simulink model "PID_controler"  (R2022b)
settings: Solver=FixedStepAuto  StartTime=0.0  StopTime=10.0  FixedStep=1e-3  MaxStep=1e-3  RelTol=1e-3
(part 2 of 2)

== system PID_controler/pid16/Subsystem2 ==
  In1 : Inport
  Derivative : Derivative
  Gain : Gain  Gain=P
  Gain1 : Gain  Gain=I
  Gain2 : Gain  Gain=D
  Integrator : Integrator
  Sum : Sum  Inputs=+++
  Out1 : Outport
  wires:
  Gain/1 -> Gain2/1, Gain1/1, Sum/1
  Gain1/1 -> Integrator/1
  Integrator/1 -> Sum/2
  Gain2/1 -> Derivative/1
  Derivative/1 -> Sum/3
  Sum/1 -> Out1/1
  In1/1 -> Gain/1

== system PID_controler/pid17/Subsystem ==
  In1 : Inport
  Derivative : Derivative
  Gain : Gain  Gain=P
  Gain1 : Gain  Gain=I
  Gain2 : Gain  Gain=D
  Integrator : Integrator
  Sum : Sum  Inputs=+++
  Out1 : Outport
  wires:
  Gain1/1 -> Integrator/1
  Gain2/1 -> Derivative/1
  Sum/1 -> Out1/1
  Integrator/1 -> Sum/2
  Gain/1 -> Sum/1
  Derivative/1 -> Sum/3
  In1/1 -> Gain/1, Gain2/1, Gain1/1

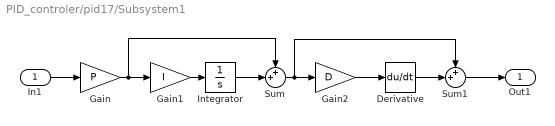
== system PID_controler/pid17/Subsystem1 ==
  In1 : Inport
  Derivative : Derivative
  Gain : Gain  Gain=P
  Gain1 : Gain  Gain=I
  Gain2 : Gain  Gain=D
  Integrator : Integrator
  Sum : Sum  Inputs=++|
  Sum1 : Sum  Inputs=++|
  Out1 : Outport
  wires:
  Sum/1 -> Sum1/1, Gain2/1
  Gain2/1 -> Derivative/1
  Gain/1 -> Sum/1, Gain1/1
  Integrator/1 -> Sum/2
  Gain1/1 -> Integrator/1
  In1/1 -> Gain/1
  Sum1/1 -> Out1/1
  Derivative/1 -> Sum1/2

== system PID_controler/pid17/Subsystem2 ==
  In1 : Inport
  Derivative : Derivative
  Gain : Gain  Gain=P
  Gain1 : Gain  Gain=I
  Gain2 : Gain  Gain=D
  Integrator : Integrator
  Sum : Sum  Inputs=+++
  Out1 : Outport
  wires:
  Gain/1 -> Gain2/1, Gain1/1, Sum/1
  Gain1/1 -> Integrator/1
  Integrator/1 -> Sum/2
  Gain2/1 -> Derivative/1
  Derivative/1 -> Sum/3
  Sum/1 -> Out1/1
  In1/1 -> Gain/1

== system PID_controler/pid18/Subsystem ==
  In1 : Inport
  Derivative : Derivative
  Gain : Gain  Gain=P
  Gain1 : Gain  Gain=I
  Gain2 : Gain  Gain=D
  Integrator : Integrator
  Sum : Sum  Inputs=+++
  Out1 : Outport
  wires:
  Gain1/1 -> Integrator/1
  Gain2/1 -> Derivative/1
  Sum/1 -> Out1/1
  Integrator/1 -> Sum/2
  Gain/1 -> Sum/1
  Derivative/1 -> Sum/3
  In1/1 -> Gain/1, Gain2/1, Gain1/1

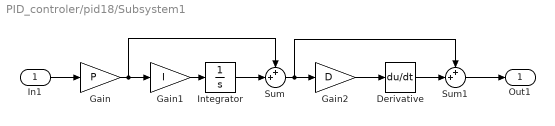
== system PID_controler/pid18/Subsystem1 ==
  In1 : Inport
  Derivative : Derivative
  Gain : Gain  Gain=P
  Gain1 : Gain  Gain=I
  Gain2 : Gain  Gain=D
  Integrator : Integrator
  Sum : Sum  Inputs=++|
  Sum1 : Sum  Inputs=++|
  Out1 : Outport
  wires:
  Sum/1 -> Sum1/1, Gain2/1
  Gain2/1 -> Derivative/1
  Gain/1 -> Sum/1, Gain1/1
  Integrator/1 -> Sum/2
  Gain1/1 -> Integrator/1
  In1/1 -> Gain/1
  Sum1/1 -> Out1/1
  Derivative/1 -> Sum1/2

== system PID_controler/pid18/Subsystem2 ==
  In1 : Inport
  Derivative : Derivative
  Gain : Gain  Gain=P
  Gain1 : Gain  Gain=I
  Gain2 : Gain  Gain=D
  Integrator : Integrator
  Sum : Sum  Inputs=+++
  Out1 : Outport
  wires:
  Gain/1 -> Gain2/1, Gain1/1, Sum/1
  Gain1/1 -> Integrator/1
  Integrator/1 -> Sum/2
  Gain2/1 -> Derivative/1
  Derivative/1 -> Sum/3
  Sum/1 -> Out1/1
  In1/1 -> Gain/1

== system PID_controler/pid19/Subsystem ==
  In1 : Inport
  Derivative : Derivative
  Gain : Gain  Gain=P
  Gain1 : Gain  Gain=I
  Gain2 : Gain  Gain=D
  Integrator : Integrator
  Sum : Sum  Inputs=+++
  Out1 : Outport
  wires:
  Gain1/1 -> Integrator/1
  Gain2/1 -> Derivative/1
  Sum/1 -> Out1/1
  Integrator/1 -> Sum/2
  Gain/1 -> Sum/1
  Derivative/1 -> Sum/3
  In1/1 -> Gain/1, Gain2/1, Gain1/1

== system PID_controler/pid19/Subsystem1 ==
  In1 : Inport
  Derivative : Derivative
  Gain : Gain  Gain=P
  Gain1 : Gain  Gain=I
  Gain2 : Gain  Gain=D
  Integrator : Integrator
  Sum : Sum  Inputs=++|
  Sum1 : Sum  Inputs=++|
  Out1 : Outport
  wires:
  Sum/1 -> Sum1/1, Gain2/1
  Gain2/1 -> Derivative/1
  Gain/1 -> Sum/1, Gain1/1
  Integrator/1 -> Sum/2
  Gain1/1 -> Integrator/1
  In1/1 -> Gain/1
  Sum1/1 -> Out1/1
  Derivative/1 -> Sum1/2

== system PID_controler/pid19/Subsystem2 ==
  In1 : Inport
  Derivative : Derivative
  Gain : Gain  Gain=P
  Gain1 : Gain  Gain=I
  Gain2 : Gain  Gain=D
  Integrator : Integrator
  Sum : Sum  Inputs=+++
  Out1 : Outport
  wires:
  Gain/1 -> Gain2/1, Gain1/1, Sum/1
  Gain1/1 -> Integrator/1
  Integrator/1 -> Sum/2
  Gain2/1 -> Derivative/1
  Derivative/1 -> Sum/3
  Sum/1 -> Out1/1
  In1/1 -> Gain/1

== system PID_controler/pid2/Subsystem ==
  In1 : Inport
  Derivative : Derivative
  Gain : Gain  Gain=P
  Gain1 : Gain  Gain=I
  Gain2 : Gain  Gain=D
  Integrator : Integrator
  Sum : Sum  Inputs=+++
  Out1 : Outport
  wires:
  In1/1 -> Gain1/1, Gain2/1, Gain/1
  Derivative/1 -> Sum/3
  Gain/1 -> Sum/1
  Integrator/1 -> Sum/2
  Sum/1 -> Out1/1
  Gain2/1 -> Derivative/1
  Gain1/1 -> Integrator/1

== system PID_controler/pid2/Subsystem1 ==
  In1 : Inport
  Derivative : Derivative
  Gain : Gain  Gain=P
  Gain1 : Gain  Gain=I
  Gain2 : Gain  Gain=D
  Integrator : Integrator
  Sum : Sum  Inputs=++|
  Sum1 : Sum  Inputs=++|
  Out1 : Outport
  wires:
  Derivative/1 -> Sum1/2
  Sum1/1 -> Out1/1
  In1/1 -> Gain/1
  Gain1/1 -> Integrator/1
  Integrator/1 -> Sum/2
  Gain/1 -> Gain1/1, Sum/1
  Gain2/1 -> Derivative/1
  Sum/1 -> Gain2/1, Sum1/1

== system PID_controler/pid2/Subsystem2 ==
  In1 : Inport
  Derivative : Derivative
  Gain : Gain  Gain=P
  Gain1 : Gain  Gain=I
  Gain2 : Gain  Gain=D
  Integrator : Integrator
  Sum : Sum  Inputs=+++
  Out1 : Outport
  wires:
  In1/1 -> Gain/1
  Sum/1 -> Out1/1
  Derivative/1 -> Sum/3
  Gain2/1 -> Derivative/1
  Integrator/1 -> Sum/2
  Gain1/1 -> Integrator/1
  Gain/1 -> Sum/1, Gain1/1, Gain2/1

== system PID_controler/pid20/Subsystem ==
  In1 : Inport
  Derivative : Derivative
  Gain : Gain  Gain=P
  Gain1 : Gain  Gain=I
  Gain2 : Gain  Gain=D
  Integrator : Integrator
  Sum : Sum  Inputs=+++
  Out1 : Outport
  wires:
  In1/1 -> Gain1/1, Gain2/1, Gain/1
  Derivative/1 -> Sum/3
  Gain/1 -> Sum/1
  Integrator/1 -> Sum/2
  Sum/1 -> Out1/1
  Gain2/1 -> Derivative/1
  Gain1/1 -> Integrator/1

== system PID_controler/pid20/Subsystem1 ==
  In1 : Inport
  Derivative : Derivative
  Gain : Gain  Gain=P
  Gain1 : Gain  Gain=I
  Gain2 : Gain  Gain=D
  Integrator : Integrator
  Sum : Sum  Inputs=++|
  Sum1 : Sum  Inputs=++|
  Out1 : Outport
  wires:
  Derivative/1 -> Sum1/2
  Sum1/1 -> Out1/1
  In1/1 -> Gain/1
  Gain1/1 -> Integrator/1
  Integrator/1 -> Sum/2
  Gain/1 -> Gain1/1, Sum/1
  Gain2/1 -> Derivative/1
  Sum/1 -> Gain2/1, Sum1/1

== system PID_controler/pid20/Subsystem2 ==
  In1 : Inport
  Derivative : Derivative
  Gain : Gain  Gain=P
  Gain1 : Gain  Gain=I
  Gain2 : Gain  Gain=D
  Integrator : Integrator
  Sum : Sum  Inputs=+++
  Out1 : Outport
  wires:
  In1/1 -> Gain/1
  Sum/1 -> Out1/1
  Derivative/1 -> Sum/3
  Gain2/1 -> Derivative/1
  Integrator/1 -> Sum/2
  Gain1/1 -> Integrator/1
  Gain/1 -> Sum/1, Gain1/1, Gain2/1

== system PID_controler/pid21/Subsystem ==
  In1 : Inport
  Derivative : Derivative
  Gain : Gain  Gain=P
  Gain1 : Gain  Gain=I
  Gain2 : Gain  Gain=D
  Integrator : Integrator
  Sum : Sum  Inputs=+++
  Out1 : Outport
  wires:
  In1/1 -> Gain1/1, Gain2/1, Gain/1
  Derivative/1 -> Sum/3
  Gain/1 -> Sum/1
  Integrator/1 -> Sum/2
  Sum/1 -> Out1/1
  Gain2/1 -> Derivative/1
  Gain1/1 -> Integrator/1

== system PID_controler/pid21/Subsystem1 ==
  In1 : Inport
  Derivative : Derivative
  Gain : Gain  Gain=P
  Gain1 : Gain  Gain=I
  Gain2 : Gain  Gain=D
  Integrator : Integrator
  Sum : Sum  Inputs=++|
  Sum1 : Sum  Inputs=++|
  Out1 : Outport
  wires:
  Derivative/1 -> Sum1/2
  Sum1/1 -> Out1/1
  In1/1 -> Gain/1
  Gain1/1 -> Integrator/1
  Integrator/1 -> Sum/2
  Gain/1 -> Gain1/1, Sum/1
  Gain2/1 -> Derivative/1
  Sum/1 -> Gain2/1, Sum1/1

== system PID_controler/pid21/Subsystem2 ==
  In1 : Inport
  Derivative : Derivative
  Gain : Gain  Gain=P
  Gain1 : Gain  Gain=I
  Gain2 : Gain  Gain=D
  Integrator : Integrator
  Sum : Sum  Inputs=+++
  Out1 : Outport
  wires:
  In1/1 -> Gain/1
  Sum/1 -> Out1/1
  Derivative/1 -> Sum/3
  Gain2/1 -> Derivative/1
  Integrator/1 -> Sum/2
  Gain1/1 -> Integrator/1
  Gain/1 -> Sum/1, Gain1/1, Gain2/1

== system PID_controler/pid22/Subsystem ==
  In1 : Inport
  Derivative : Derivative
  Gain : Gain  Gain=P
  Gain1 : Gain  Gain=I
  Gain2 : Gain  Gain=D
  Integrator : Integrator
  Sum : Sum  Inputs=+++
  Out1 : Outport
  wires:
  In1/1 -> Gain1/1, Gain2/1, Gain/1
  Derivative/1 -> Sum/3
  Gain/1 -> Sum/1
  Integrator/1 -> Sum/2
  Sum/1 -> Out1/1
  Gain2/1 -> Derivative/1
  Gain1/1 -> Integrator/1

== system PID_controler/pid22/Subsystem1 ==
  In1 : Inport
  Derivative : Derivative
  Gain : Gain  Gain=P
  Gain1 : Gain  Gain=I
  Gain2 : Gain  Gain=D
  Integrator : Integrator
  Sum : Sum  Inputs=++|
  Sum1 : Sum  Inputs=++|
  Out1 : Outport
  wires:
  Derivative/1 -> Sum1/2
  Sum1/1 -> Out1/1
  In1/1 -> Gain/1
  Gain1/1 -> Integrator/1
  Integrator/1 -> Sum/2
  Gain/1 -> Gain1/1, Sum/1
  Gain2/1 -> Derivative/1
  Sum/1 -> Gain2/1, Sum1/1

== system PID_controler/pid22/Subsystem2 ==
  In1 : Inport
  Derivative : Derivative
  Gain : Gain  Gain=P
  Gain1 : Gain  Gain=I
  Gain2 : Gain  Gain=D
  Integrator : Integrator
  Sum : Sum  Inputs=+++
  Out1 : Outport
  wires:
  In1/1 -> Gain/1
  Sum/1 -> Out1/1
  Derivative/1 -> Sum/3
  Gain2/1 -> Derivative/1
  Integrator/1 -> Sum/2
  Gain1/1 -> Integrator/1
  Gain/1 -> Sum/1, Gain1/1, Gain2/1

== system PID_controler/pid23/Subsystem ==
  In1 : Inport
  Derivative : Derivative
  Gain : Gain  Gain=P
  Gain1 : Gain  Gain=I
  Gain2 : Gain  Gain=D
  Integrator : Integrator
  Sum : Sum  Inputs=+++
  Out1 : Outport
  wires:
  In1/1 -> Gain1/1, Gain2/1, Gain/1
  Derivative/1 -> Sum/3
  Gain/1 -> Sum/1
  Integrator/1 -> Sum/2
  Sum/1 -> Out1/1
  Gain2/1 -> Derivative/1
  Gain1/1 -> Integrator/1

== system PID_controler/pid23/Subsystem1 ==
  In1 : Inport
  Derivative : Derivative
  Gain : Gain  Gain=P
  Gain1 : Gain  Gain=I
  Gain2 : Gain  Gain=D
  Integrator : Integrator
  Sum : Sum  Inputs=++|
  Sum1 : Sum  Inputs=++|
  Out1 : Outport
  wires:
  Derivative/1 -> Sum1/2
  Sum1/1 -> Out1/1
  In1/1 -> Gain/1
  Gain1/1 -> Integrator/1
  Integrator/1 -> Sum/2
  Gain/1 -> Gain1/1, Sum/1
  Gain2/1 -> Derivative/1
  Sum/1 -> Gain2/1, Sum1/1

== system PID_controler/pid23/Subsystem2 ==
  In1 : Inport
  Derivative : Derivative
  Gain : Gain  Gain=P
  Gain1 : Gain  Gain=I
  Gain2 : Gain  Gain=D
  Integrator : Integrator
  Sum : Sum  Inputs=+++
  Out1 : Outport
  wires:
  In1/1 -> Gain/1
  Sum/1 -> Out1/1
  Derivative/1 -> Sum/3
  Gain2/1 -> Derivative/1
  Integrator/1 -> Sum/2
  Gain1/1 -> Integrator/1
  Gain/1 -> Sum/1, Gain1/1, Gain2/1

== system PID_controler/pid24/Subsystem ==
  In1 : Inport
  Derivative : Derivative
  Gain : Gain  Gain=P
  Gain1 : Gain  Gain=I
  Gain2 : Gain  Gain=D
  Integrator : Integrator
  Sum : Sum  Inputs=+++
  Out1 : Outport
  wires:
  In1/1 -> Gain1/1, Gain2/1, Gain/1
  Derivative/1 -> Sum/3
  Gain/1 -> Sum/1
  Integrator/1 -> Sum/2
  Sum/1 -> Out1/1
  Gain2/1 -> Derivative/1
  Gain1/1 -> Integrator/1

== system PID_controler/pid24/Subsystem1 ==
  In1 : Inport
  Derivative : Derivative
  Gain : Gain  Gain=P
  Gain1 : Gain  Gain=I
  Gain2 : Gain  Gain=D
  Integrator : Integrator
  Sum : Sum  Inputs=++|
  Sum1 : Sum  Inputs=++|
  Out1 : Outport
  wires:
  Derivative/1 -> Sum1/2
  Sum1/1 -> Out1/1
  In1/1 -> Gain/1
  Gain1/1 -> Integrator/1
  Integrator/1 -> Sum/2
  Gain/1 -> Gain1/1, Sum/1
  Gain2/1 -> Derivative/1
  Sum/1 -> Gain2/1, Sum1/1

== system PID_controler/pid24/Subsystem2 ==
  In1 : Inport
  Derivative : Derivative
  Gain : Gain  Gain=P
  Gain1 : Gain  Gain=I
  Gain2 : Gain  Gain=D
  Integrator : Integrator
  Sum : Sum  Inputs=+++
  Out1 : Outport
  wires:
  In1/1 -> Gain/1
  Sum/1 -> Out1/1
  Derivative/1 -> Sum/3
  Gain2/1 -> Derivative/1
  Integrator/1 -> Sum/2
  Gain1/1 -> Integrator/1
  Gain/1 -> Sum/1, Gain1/1, Gain2/1

== system PID_controler/pid25/Subsystem ==
  In1 : Inport
  Derivative : Derivative
  Gain : Gain  Gain=P
  Gain1 : Gain  Gain=I
  Gain2 : Gain  Gain=D
  Integrator : Integrator
  Sum : Sum  Inputs=+++
  Out1 : Outport
  wires:
  In1/1 -> Gain1/1, Gain2/1, Gain/1
  Derivative/1 -> Sum/3
  Gain/1 -> Sum/1
  Integrator/1 -> Sum/2
  Sum/1 -> Out1/1
  Gain2/1 -> Derivative/1
  Gain1/1 -> Integrator/1

== system PID_controler/pid25/Subsystem1 ==
  In1 : Inport
  Derivative : Derivative
  Gain : Gain  Gain=P
  Gain1 : Gain  Gain=I
  Gain2 : Gain  Gain=D
  Integrator : Integrator
  Sum : Sum  Inputs=++|
  Sum1 : Sum  Inputs=++|
  Out1 : Outport
  wires:
  Derivative/1 -> Sum1/2
  Sum1/1 -> Out1/1
  In1/1 -> Gain/1
  Gain1/1 -> Integrator/1
  Integrator/1 -> Sum/2
  Gain/1 -> Gain1/1, Sum/1
  Gain2/1 -> Derivative/1
  Sum/1 -> Gain2/1, Sum1/1

== system PID_controler/pid25/Subsystem2 ==
  In1 : Inport
  Derivative : Derivative
  Gain : Gain  Gain=P
  Gain1 : Gain  Gain=I
  Gain2 : Gain  Gain=D
  Integrator : Integrator
  Sum : Sum  Inputs=+++
  Out1 : Outport
  wires:
  In1/1 -> Gain/1
  Sum/1 -> Out1/1
  Derivative/1 -> Sum/3
  Gain2/1 -> Derivative/1
  Integrator/1 -> Sum/2
  Gain1/1 -> Integrator/1
  Gain/1 -> Sum/1, Gain1/1, Gain2/1

== system PID_controler/pid26/Subsystem ==
  In1 : Inport
  Derivative : Derivative
  Gain : Gain  Gain=P
  Gain1 : Gain  Gain=I
  Gain2 : Gain  Gain=D
  Integrator : Integrator
  Sum : Sum  Inputs=+++
  Out1 : Outport
  wires:
  In1/1 -> Gain1/1, Gain2/1, Gain/1
  Derivative/1 -> Sum/3
  Gain/1 -> Sum/1
  Integrator/1 -> Sum/2
  Sum/1 -> Out1/1
  Gain2/1 -> Derivative/1
  Gain1/1 -> Integrator/1

== system PID_controler/pid26/Subsystem1 ==
  In1 : Inport
  Derivative : Derivative
  Gain : Gain  Gain=P
  Gain1 : Gain  Gain=I
  Gain2 : Gain  Gain=D
  Integrator : Integrator
  Sum : Sum  Inputs=++|
  Sum1 : Sum  Inputs=++|
  Out1 : Outport
  wires:
  Derivative/1 -> Sum1/2
  Sum1/1 -> Out1/1
  In1/1 -> Gain/1
  Gain1/1 -> Integrator/1
  Integrator/1 -> Sum/2
  Gain/1 -> Gain1/1, Sum/1
  Gain2/1 -> Derivative/1
  Sum/1 -> Gain2/1, Sum1/1

== system PID_controler/pid26/Subsystem2 ==
  In1 : Inport
  Derivative : Derivative
  Gain : Gain  Gain=P
  Gain1 : Gain  Gain=I
  Gain2 : Gain  Gain=D
  Integrator : Integrator
  Sum : Sum  Inputs=+++
  Out1 : Outport
  wires:
  In1/1 -> Gain/1
  Sum/1 -> Out1/1
  Derivative/1 -> Sum/3
  Gain2/1 -> Derivative/1
  Integrator/1 -> Sum/2
  Gain1/1 -> Integrator/1
  Gain/1 -> Sum/1, Gain1/1, Gain2/1

== system PID_controler/pid27/Subsystem ==
  In1 : Inport
  Derivative : Derivative
  Gain : Gain  Gain=P
  Gain1 : Gain  Gain=I
  Gain2 : Gain  Gain=D
  Integrator : Integrator
  Sum : Sum  Inputs=+++
  Out1 : Outport
  wires:
  In1/1 -> Gain1/1, Gain2/1, Gain/1
  Derivative/1 -> Sum/3
  Gain/1 -> Sum/1
  Integrator/1 -> Sum/2
  Sum/1 -> Out1/1
  Gain2/1 -> Derivative/1
  Gain1/1 -> Integrator/1

== system PID_controler/pid27/Subsystem1 ==
  In1 : Inport
  Derivative : Derivative
  Gain : Gain  Gain=P
  Gain1 : Gain  Gain=I
  Gain2 : Gain  Gain=D
  Integrator : Integrator
  Sum : Sum  Inputs=++|
  Sum1 : Sum  Inputs=++|
  Out1 : Outport
  wires:
  Derivative/1 -> Sum1/2
  Sum1/1 -> Out1/1
  In1/1 -> Gain/1
  Gain1/1 -> Integrator/1
  Integrator/1 -> Sum/2
  Gain/1 -> Gain1/1, Sum/1
  Gain2/1 -> Derivative/1
  Sum/1 -> Gain2/1, Sum1/1

== system PID_controler/pid27/Subsystem2 ==
  In1 : Inport
  Derivative : Derivative
  Gain : Gain  Gain=P
  Gain1 : Gain  Gain=I
  Gain2 : Gain  Gain=D
  Integrator : Integrator
  Sum : Sum  Inputs=+++
  Out1 : Outport
  wires:
  In1/1 -> Gain/1
  Sum/1 -> Out1/1
  Derivative/1 -> Sum/3
  Gain2/1 -> Derivative/1
  Integrator/1 -> Sum/2
  Gain1/1 -> Integrator/1
  Gain/1 -> Sum/1, Gain1/1, Gain2/1

== system PID_controler/pid28/Subsystem ==
  In1 : Inport
  Derivative : Derivative
  Gain : Gain  Gain=P
  Gain1 : Gain  Gain=I
  Gain2 : Gain  Gain=D
  Integrator : Integrator
  Sum : Sum  Inputs=+++
  Out1 : Outport
  wires:
  In1/1 -> Gain1/1, Gain2/1, Gain/1
  Derivative/1 -> Sum/3
  Gain/1 -> Sum/1
  Integrator/1 -> Sum/2
  Sum/1 -> Out1/1
  Gain2/1 -> Derivative/1
  Gain1/1 -> Integrator/1

== system PID_controler/pid28/Subsystem1 ==
  In1 : Inport
  Derivative : Derivative
  Gain : Gain  Gain=P
  Gain1 : Gain  Gain=I
  Gain2 : Gain  Gain=D
  Integrator : Integrator
  Sum : Sum  Inputs=++|
  Sum1 : Sum  Inputs=++|
  Out1 : Outport
  wires:
  Derivative/1 -> Sum1/2
  Sum1/1 -> Out1/1
  In1/1 -> Gain/1
  Gain1/1 -> Integrator/1
  Integrator/1 -> Sum/2
  Gain/1 -> Gain1/1, Sum/1
  Gain2/1 -> Derivative/1
  Sum/1 -> Gain2/1, Sum1/1

== system PID_controler/pid28/Subsystem2 ==
  In1 : Inport
  Derivative : Derivative
  Gain : Gain  Gain=P
  Gain1 : Gain  Gain=I
  Gain2 : Gain  Gain=D
  Integrator : Integrator
  Sum : Sum  Inputs=+++
  Out1 : Outport
  wires:
  In1/1 -> Gain/1
  Sum/1 -> Out1/1
  Derivative/1 -> Sum/3
  Gain2/1 -> Derivative/1
  Integrator/1 -> Sum/2
  Gain1/1 -> Integrator/1
  Gain/1 -> Sum/1, Gain1/1, Gain2/1

== system PID_controler/pid29/Subsystem ==
  In1 : Inport
  Derivative : Derivative
  Gain : Gain  Gain=P
  Gain1 : Gain  Gain=I
  Gain2 : Gain  Gain=D
  Integrator : Integrator
  Sum : Sum  Inputs=+++
  Out1 : Outport
  wires:
  In1/1 -> Gain1/1, Gain2/1, Gain/1
  Derivative/1 -> Sum/3
  Gain/1 -> Sum/1
  Integrator/1 -> Sum/2
  Sum/1 -> Out1/1
  Gain2/1 -> Derivative/1
  Gain1/1 -> Integrator/1

== system PID_controler/pid29/Subsystem1 ==
  In1 : Inport
  Derivative : Derivative
  Gain : Gain  Gain=P
  Gain1 : Gain  Gain=I
  Gain2 : Gain  Gain=D
  Integrator : Integrator
  Sum : Sum  Inputs=++|
  Sum1 : Sum  Inputs=++|
  Out1 : Outport
  wires:
  Derivative/1 -> Sum1/2
  Sum1/1 -> Out1/1
  In1/1 -> Gain/1
  Gain1/1 -> Integrator/1
  Integrator/1 -> Sum/2
  Gain/1 -> Gain1/1, Sum/1
  Gain2/1 -> Derivative/1
  Sum/1 -> Gain2/1, Sum1/1

== system PID_controler/pid29/Subsystem2 ==
  In1 : Inport
  Derivative : Derivative
  Gain : Gain  Gain=P
  Gain1 : Gain  Gain=I
  Gain2 : Gain  Gain=D
  Integrator : Integrator
  Sum : Sum  Inputs=+++
  Out1 : Outport
  wires:
  In1/1 -> Gain/1
  Sum/1 -> Out1/1
  Derivative/1 -> Sum/3
  Gain2/1 -> Derivative/1
  Integrator/1 -> Sum/2
  Gain1/1 -> Integrator/1
  Gain/1 -> Sum/1, Gain1/1, Gain2/1

== system PID_controler/pid3/Subsystem ==
  In1 : Inport
  Derivative : Derivative
  Gain : Gain  Gain=P
  Gain1 : Gain  Gain=I
  Gain2 : Gain  Gain=D
  Integrator : Integrator
  Sum : Sum  Inputs=+++
  Out1 : Outport
  wires:
  In1/1 -> Gain1/1, Gain2/1, Gain/1
  Derivative/1 -> Sum/3
  Gain/1 -> Sum/1
  Integrator/1 -> Sum/2
  Sum/1 -> Out1/1
  Gain2/1 -> Derivative/1
  Gain1/1 -> Integrator/1

== system PID_controler/pid3/Subsystem1 ==
  In1 : Inport
  Derivative : Derivative
  Gain : Gain  Gain=P
  Gain1 : Gain  Gain=I
  Gain2 : Gain  Gain=D
  Integrator : Integrator
  Sum : Sum  Inputs=++|
  Sum1 : Sum  Inputs=++|
  Out1 : Outport
  wires:
  Derivative/1 -> Sum1/2
  Sum1/1 -> Out1/1
  In1/1 -> Gain/1
  Gain1/1 -> Integrator/1
  Integrator/1 -> Sum/2
  Gain/1 -> Gain1/1, Sum/1
  Gain2/1 -> Derivative/1
  Sum/1 -> Gain2/1, Sum1/1

== system PID_controler/pid3/Subsystem2 ==
  In1 : Inport
  Derivative : Derivative
  Gain : Gain  Gain=P
  Gain1 : Gain  Gain=I
  Gain2 : Gain  Gain=D
  Integrator : Integrator
  Sum : Sum  Inputs=+++
  Out1 : Outport
  wires:
  In1/1 -> Gain/1
  Sum/1 -> Out1/1
  Derivative/1 -> Sum/3
  Gain2/1 -> Derivative/1
  Integrator/1 -> Sum/2
  Gain1/1 -> Integrator/1
  Gain/1 -> Sum/1, Gain1/1, Gain2/1

== system PID_controler/pid30/Subsystem ==
  In1 : Inport
  Derivative : Derivative
  Gain : Gain  Gain=P
  Gain1 : Gain  Gain=I
  Gain2 : Gain  Gain=D
  Integrator : Integrator
  Sum : Sum  Inputs=+++
  Out1 : Outport
  wires:
  Gain1/1 -> Integrator/1
  Gain2/1 -> Derivative/1
  Sum/1 -> Out1/1
  Integrator/1 -> Sum/2
  Gain/1 -> Sum/1
  Derivative/1 -> Sum/3
  In1/1 -> Gain/1, Gain2/1, Gain1/1

== system PID_controler/pid30/Subsystem1 ==
  In1 : Inport
  Derivative : Derivative
  Gain : Gain  Gain=P
  Gain1 : Gain  Gain=I
  Gain2 : Gain  Gain=D
  Integrator : Integrator
  Sum : Sum  Inputs=++|
  Sum1 : Sum  Inputs=++|
  Out1 : Outport
  wires:
  Sum/1 -> Sum1/1, Gain2/1
  Gain2/1 -> Derivative/1
  Gain/1 -> Sum/1, Gain1/1
  Integrator/1 -> Sum/2
  Gain1/1 -> Integrator/1
  In1/1 -> Gain/1
  Sum1/1 -> Out1/1
  Derivative/1 -> Sum1/2

== system PID_controler/pid30/Subsystem2 ==
  In1 : Inport
  Derivative : Derivative
  Gain : Gain  Gain=P
  Gain1 : Gain  Gain=I
  Gain2 : Gain  Gain=D
  Integrator : Integrator
  Sum : Sum  Inputs=+++
  Out1 : Outport
  wires:
  Gain/1 -> Gain2/1, Gain1/1, Sum/1
  Gain1/1 -> Integrator/1
  Integrator/1 -> Sum/2
  Gain2/1 -> Derivative/1
  Derivative/1 -> Sum/3
  Sum/1 -> Out1/1
  In1/1 -> Gain/1

== system PID_controler/pid31/Subsystem ==
  In1 : Inport
  Derivative : Derivative
  Gain : Gain  Gain=P
  Gain1 : Gain  Gain=I
  Gain2 : Gain  Gain=D
  Integrator : Integrator
  Sum : Sum  Inputs=+++
  Out1 : Outport
  wires:
  Gain1/1 -> Integrator/1
  Gain2/1 -> Derivative/1
  Sum/1 -> Out1/1
  Integrator/1 -> Sum/2
  Gain/1 -> Sum/1
  Derivative/1 -> Sum/3
  In1/1 -> Gain/1, Gain2/1, Gain1/1

== system PID_controler/pid31/Subsystem1 ==
  In1 : Inport
  Derivative : Derivative
  Gain : Gain  Gain=P
  Gain1 : Gain  Gain=I
  Gain2 : Gain  Gain=D
  Integrator : Integrator
  Sum : Sum  Inputs=++|
  Sum1 : Sum  Inputs=++|
  Out1 : Outport
  wires:
  Sum/1 -> Sum1/1, Gain2/1
  Gain2/1 -> Derivative/1
  Gain/1 -> Sum/1, Gain1/1
  Integrator/1 -> Sum/2
  Gain1/1 -> Integrator/1
  In1/1 -> Gain/1
  Sum1/1 -> Out1/1
  Derivative/1 -> Sum1/2

== system PID_controler/pid31/Subsystem2 ==
  In1 : Inport
  Derivative : Derivative
  Gain : Gain  Gain=P
  Gain1 : Gain  Gain=I
  Gain2 : Gain  Gain=D
  Integrator : Integrator
  Sum : Sum  Inputs=+++
  Out1 : Outport
  wires:
  Gain/1 -> Gain2/1, Gain1/1, Sum/1
  Gain1/1 -> Integrator/1
  Integrator/1 -> Sum/2
  Gain2/1 -> Derivative/1
  Derivative/1 -> Sum/3
  Sum/1 -> Out1/1
  In1/1 -> Gain/1

== system PID_controler/pid32/Subsystem ==
  In1 : Inport
  Derivative : Derivative
  Gain : Gain  Gain=P
  Gain1 : Gain  Gain=I
  Gain2 : Gain  Gain=D
  Integrator : Integrator
  Sum : Sum  Inputs=+++
  Out1 : Outport
  wires:
  Gain1/1 -> Integrator/1
  Gain2/1 -> Derivative/1
  Sum/1 -> Out1/1
  Integrator/1 -> Sum/2
  Gain/1 -> Sum/1
  Derivative/1 -> Sum/3
  In1/1 -> Gain/1, Gain2/1, Gain1/1

== system PID_controler/pid32/Subsystem1 ==
  In1 : Inport
  Derivative : Derivative
  Gain : Gain  Gain=P
  Gain1 : Gain  Gain=I
  Gain2 : Gain  Gain=D
  Integrator : Integrator
  Sum : Sum  Inputs=++|
  Sum1 : Sum  Inputs=++|
  Out1 : Outport
  wires:
  Sum/1 -> Sum1/1, Gain2/1
  Gain2/1 -> Derivative/1
  Gain/1 -> Sum/1, Gain1/1
  Integrator/1 -> Sum/2
  Gain1/1 -> Integrator/1
  In1/1 -> Gain/1
  Sum1/1 -> Out1/1
  Derivative/1 -> Sum1/2

== system PID_controler/pid32/Subsystem2 ==
  In1 : Inport
  Derivative : Derivative
  Gain : Gain  Gain=P
  Gain1 : Gain  Gain=I
  Gain2 : Gain  Gain=D
  Integrator : Integrator
  Sum : Sum  Inputs=+++
  Out1 : Outport
  wires:
  Gain/1 -> Gain2/1, Gain1/1, Sum/1
  Gain1/1 -> Integrator/1
  Integrator/1 -> Sum/2
  Gain2/1 -> Derivative/1
  Derivative/1 -> Sum/3
  Sum/1 -> Out1/1
  In1/1 -> Gain/1

== system PID_controler/pid33/Subsystem ==
  In1 : Inport
  Derivative : Derivative
  Gain : Gain  Gain=P
  Gain1 : Gain  Gain=I
  Gain2 : Gain  Gain=D
  Integrator : Integrator
  Sum : Sum  Inputs=+++
  Out1 : Outport
  wires:
  Gain1/1 -> Integrator/1
  Gain2/1 -> Derivative/1
  Sum/1 -> Out1/1
  Integrator/1 -> Sum/2
  Gain/1 -> Sum/1
  Derivative/1 -> Sum/3
  In1/1 -> Gain/1, Gain2/1, Gain1/1

== system PID_controler/pid33/Subsystem1 ==
  In1 : Inport
  Derivative : Derivative
  Gain : Gain  Gain=P
  Gain1 : Gain  Gain=I
  Gain2 : Gain  Gain=D
  Integrator : Integrator
  Sum : Sum  Inputs=++|
  Sum1 : Sum  Inputs=++|
  Out1 : Outport
  wires:
  Sum/1 -> Sum1/1, Gain2/1
  Gain2/1 -> Derivative/1
  Gain/1 -> Sum/1, Gain1/1
  Integrator/1 -> Sum/2
  Gain1/1 -> Integrator/1
  In1/1 -> Gain/1
  Sum1/1 -> Out1/1
  Derivative/1 -> Sum1/2

== system PID_controler/pid33/Subsystem2 ==
  In1 : Inport
  Derivative : Derivative
  Gain : Gain  Gain=P
  Gain1 : Gain  Gain=I
  Gain2 : Gain  Gain=D
  Integrator : Integrator
  Sum : Sum  Inputs=+++
  Out1 : Outport
  wires:
  Gain/1 -> Gain2/1, Gain1/1, Sum/1
  Gain1/1 -> Integrator/1
  Integrator/1 -> Sum/2
  Gain2/1 -> Derivative/1
  Derivative/1 -> Sum/3
  Sum/1 -> Out1/1
  In1/1 -> Gain/1

== system PID_controler/pid34/Subsystem ==
  In1 : Inport
  Derivative : Derivative
  Gain : Gain  Gain=P
  Gain1 : Gain  Gain=I
  Gain2 : Gain  Gain=D
  Integrator : Integrator
  Sum : Sum  Inputs=+++
  Out1 : Outport
  wires:
  Gain1/1 -> Integrator/1
  Gain2/1 -> Derivative/1
  Sum/1 -> Out1/1
  Integrator/1 -> Sum/2
  Gain/1 -> Sum/1
  Derivative/1 -> Sum/3
  In1/1 -> Gain/1, Gain2/1, Gain1/1

== system PID_controler/pid34/Subsystem1 ==
  In1 : Inport
  Derivative : Derivative
  Gain : Gain  Gain=P
  Gain1 : Gain  Gain=I
  Gain2 : Gain  Gain=D
  Integrator : Integrator
  Sum : Sum  Inputs=++|
  Sum1 : Sum  Inputs=++|
  Out1 : Outport
  wires:
  Sum/1 -> Sum1/1, Gain2/1
  Gain2/1 -> Derivative/1
  Gain/1 -> Sum/1, Gain1/1
  Integrator/1 -> Sum/2
  Gain1/1 -> Integrator/1
  In1/1 -> Gain/1
  Sum1/1 -> Out1/1
  Derivative/1 -> Sum1/2

== system PID_controler/pid34/Subsystem2 ==
  In1 : Inport
  Derivative : Derivative
  Gain : Gain  Gain=P
  Gain1 : Gain  Gain=I
  Gain2 : Gain  Gain=D
  Integrator : Integrator
  Sum : Sum  Inputs=+++
  Out1 : Outport
  wires:
  Gain/1 -> Gain2/1, Gain1/1, Sum/1
  Gain1/1 -> Integrator/1
  Integrator/1 -> Sum/2
  Gain2/1 -> Derivative/1
  Derivative/1 -> Sum/3
  Sum/1 -> Out1/1
  In1/1 -> Gain/1

== system PID_controler/pid4/Subsystem ==
  In1 : Inport
  Derivative : Derivative
  Gain : Gain  Gain=P
  Gain1 : Gain  Gain=I
  Gain2 : Gain  Gain=D
  Integrator : Integrator
  Sum : Sum  Inputs=+++
  Out1 : Outport
  wires:
  In1/1 -> Gain1/1, Gain2/1, Gain/1
  Derivative/1 -> Sum/3
  Gain/1 -> Sum/1
  Integrator/1 -> Sum/2
  Sum/1 -> Out1/1
  Gain2/1 -> Derivative/1
  Gain1/1 -> Integrator/1

== system PID_controler/pid4/Subsystem1 ==
  In1 : Inport
  Derivative : Derivative
  Gain : Gain  Gain=P
  Gain1 : Gain  Gain=I
  Gain2 : Gain  Gain=D
  Integrator : Integrator
  Sum : Sum  Inputs=++|
  Sum1 : Sum  Inputs=++|
  Out1 : Outport
  wires:
  Derivative/1 -> Sum1/2
  Sum1/1 -> Out1/1
  In1/1 -> Gain/1
  Gain1/1 -> Integrator/1
  Integrator/1 -> Sum/2
  Gain/1 -> Gain1/1, Sum/1
  Gain2/1 -> Derivative/1
  Sum/1 -> Gain2/1, Sum1/1

== system PID_controler/pid4/Subsystem2 ==
  In1 : Inport
  Derivative : Derivative
  Gain : Gain  Gain=P
  Gain1 : Gain  Gain=I
  Gain2 : Gain  Gain=D
  Integrator : Integrator
  Sum : Sum  Inputs=+++
  Out1 : Outport
  wires:
  In1/1 -> Gain/1
  Sum/1 -> Out1/1
  Derivative/1 -> Sum/3
  Gain2/1 -> Derivative/1
  Integrator/1 -> Sum/2
  Gain1/1 -> Integrator/1
  Gain/1 -> Sum/1, Gain1/1, Gain2/1

== system PID_controler/pid5/Subsystem ==
  In1 : Inport
  Derivative : Derivative
  Gain : Gain  Gain=P
  Gain1 : Gain  Gain=I
  Gain2 : Gain  Gain=D
  Integrator : Integrator
  Sum : Sum  Inputs=+++
  Out1 : Outport
  wires:
  In1/1 -> Gain1/1, Gain2/1, Gain/1
  Derivative/1 -> Sum/3
  Gain/1 -> Sum/1
  Integrator/1 -> Sum/2
  Sum/1 -> Out1/1
  Gain2/1 -> Derivative/1
  Gain1/1 -> Integrator/1

== system PID_controler/pid5/Subsystem1 ==
  In1 : Inport
  Derivative : Derivative
  Gain : Gain  Gain=P
  Gain1 : Gain  Gain=I
  Gain2 : Gain  Gain=D
  Integrator : Integrator
  Sum : Sum  Inputs=++|
  Sum1 : Sum  Inputs=++|
  Out1 : Outport
  wires:
  Derivative/1 -> Sum1/2
  Sum1/1 -> Out1/1
  In1/1 -> Gain/1
  Gain1/1 -> Integrator/1
  Integrator/1 -> Sum/2
  Gain/1 -> Gain1/1, Sum/1
  Gain2/1 -> Derivative/1
  Sum/1 -> Gain2/1, Sum1/1

== system PID_controler/pid5/Subsystem2 ==
  In1 : Inport
  Derivative : Derivative
  Gain : Gain  Gain=P
  Gain1 : Gain  Gain=I
  Gain2 : Gain  Gain=D
  Integrator : Integrator
  Sum : Sum  Inputs=+++
  Out1 : Outport
  wires:
  In1/1 -> Gain/1
  Sum/1 -> Out1/1
  Derivative/1 -> Sum/3
  Gain2/1 -> Derivative/1
  Integrator/1 -> Sum/2
  Gain1/1 -> Integrator/1
  Gain/1 -> Sum/1, Gain1/1, Gain2/1

== system PID_controler/pid6/Subsystem ==
  In1 : Inport
  Derivative : Derivative
  Gain : Gain  Gain=P
  Gain1 : Gain  Gain=I
  Gain2 : Gain  Gain=D
  Integrator : Integrator
  Sum : Sum  Inputs=+++
  Out1 : Outport
  wires:
  In1/1 -> Gain1/1, Gain2/1, Gain/1
  Derivative/1 -> Sum/3
  Gain/1 -> Sum/1
  Integrator/1 -> Sum/2
  Sum/1 -> Out1/1
  Gain2/1 -> Derivative/1
  Gain1/1 -> Integrator/1

== system PID_controler/pid6/Subsystem1 ==
  In1 : Inport
  Derivative : Derivative
  Gain : Gain  Gain=P
  Gain1 : Gain  Gain=I
  Gain2 : Gain  Gain=D
  Integrator : Integrator
  Sum : Sum  Inputs=++|
  Sum1 : Sum  Inputs=++|
  Out1 : Outport
  wires:
  Derivative/1 -> Sum1/2
  Sum1/1 -> Out1/1
  In1/1 -> Gain/1
  Gain1/1 -> Integrator/1
  Integrator/1 -> Sum/2
  Gain/1 -> Gain1/1, Sum/1
  Gain2/1 -> Derivative/1
  Sum/1 -> Gain2/1, Sum1/1

== system PID_controler/pid6/Subsystem2 ==
  In1 : Inport
  Derivative : Derivative
  Gain : Gain  Gain=P
  Gain1 : Gain  Gain=I
  Gain2 : Gain  Gain=D
  Integrator : Integrator
  Sum : Sum  Inputs=+++
  Out1 : Outport
  wires:
  In1/1 -> Gain/1
  Sum/1 -> Out1/1
  Derivative/1 -> Sum/3
  Gain2/1 -> Derivative/1
  Integrator/1 -> Sum/2
  Gain1/1 -> Integrator/1
  Gain/1 -> Sum/1, Gain1/1, Gain2/1

== system PID_controler/pid7/Subsystem ==
  In1 : Inport
  Derivative : Derivative
  Gain : Gain  Gain=P
  Gain1 : Gain  Gain=I
  Gain2 : Gain  Gain=D
  Integrator : Integrator
  Sum : Sum  Inputs=+++
  Out1 : Outport
  wires:
  In1/1 -> Gain1/1, Gain2/1, Gain/1
  Derivative/1 -> Sum/3
  Gain/1 -> Sum/1
  Integrator/1 -> Sum/2
  Sum/1 -> Out1/1
  Gain2/1 -> Derivative/1
  Gain1/1 -> Integrator/1

== system PID_controler/pid7/Subsystem1 ==
  In1 : Inport
  Derivative : Derivative
  Gain : Gain  Gain=P
  Gain1 : Gain  Gain=I
  Gain2 : Gain  Gain=D
  Integrator : Integrator
  Sum : Sum  Inputs=++|
  Sum1 : Sum  Inputs=++|
  Out1 : Outport
  wires:
  Derivative/1 -> Sum1/2
  Sum1/1 -> Out1/1
  In1/1 -> Gain/1
  Gain1/1 -> Integrator/1
  Integrator/1 -> Sum/2
  Gain/1 -> Gain1/1, Sum/1
  Gain2/1 -> Derivative/1
  Sum/1 -> Gain2/1, Sum1/1

== system PID_controler/pid7/Subsystem2 ==
  In1 : Inport
  Derivative : Derivative
  Gain : Gain  Gain=P
  Gain1 : Gain  Gain=I
  Gain2 : Gain  Gain=D
  Integrator : Integrator
  Sum : Sum  Inputs=+++
  Out1 : Outport
  wires:
  In1/1 -> Gain/1
  Sum/1 -> Out1/1
  Derivative/1 -> Sum/3
  Gain2/1 -> Derivative/1
  Integrator/1 -> Sum/2
  Gain1/1 -> Integrator/1
  Gain/1 -> Sum/1, Gain1/1, Gain2/1

== system PID_controler/pid8/Subsystem ==
  In1 : Inport
  Derivative : Derivative
  Gain : Gain  Gain=P
  Gain1 : Gain  Gain=I
  Gain2 : Gain  Gain=D
  Integrator : Integrator
  Sum : Sum  Inputs=+++
  Out1 : Outport
  wires:
  In1/1 -> Gain1/1, Gain2/1, Gain/1
  Derivative/1 -> Sum/3
  Gain/1 -> Sum/1
  Integrator/1 -> Sum/2
  Sum/1 -> Out1/1
  Gain2/1 -> Derivative/1
  Gain1/1 -> Integrator/1

== system PID_controler/pid8/Subsystem1 ==
  In1 : Inport
  Derivative : Derivative
  Gain : Gain  Gain=P
  Gain1 : Gain  Gain=I
  Gain2 : Gain  Gain=D
  Integrator : Integrator
  Sum : Sum  Inputs=++|
  Sum1 : Sum  Inputs=++|
  Out1 : Outport
  wires:
  Derivative/1 -> Sum1/2
  Sum1/1 -> Out1/1
  In1/1 -> Gain/1
  Gain1/1 -> Integrator/1
  Integrator/1 -> Sum/2
  Gain/1 -> Gain1/1, Sum/1
  Gain2/1 -> Derivative/1
  Sum/1 -> Gain2/1, Sum1/1

== system PID_controler/pid8/Subsystem2 ==
  In1 : Inport
  Derivative : Derivative
  Gain : Gain  Gain=P
  Gain1 : Gain  Gain=I
  Gain2 : Gain  Gain=D
  Integrator : Integrator
  Sum : Sum  Inputs=+++
  Out1 : Outport
  wires:
  In1/1 -> Gain/1
  Sum/1 -> Out1/1
  Derivative/1 -> Sum/3
  Gain2/1 -> Derivative/1
  Integrator/1 -> Sum/2
  Gain1/1 -> Integrator/1
  Gain/1 -> Sum/1, Gain1/1, Gain2/1

== system PID_controler/pid9/Subsystem ==
  In1 : Inport
  Derivative : Derivative
  Gain : Gain  Gain=P
  Gain1 : Gain  Gain=I
  Gain2 : Gain  Gain=D
  Integrator : Integrator
  Sum : Sum  Inputs=+++
  Out1 : Outport
  wires:
  In1/1 -> Gain1/1, Gain2/1, Gain/1
  Derivative/1 -> Sum/3
  Gain/1 -> Sum/1
  Integrator/1 -> Sum/2
  Sum/1 -> Out1/1
  Gain2/1 -> Derivative/1
  Gain1/1 -> Integrator/1

== system PID_controler/pid9/Subsystem1 ==
  In1 : Inport
  Derivative : Derivative
  Gain : Gain  Gain=P
  Gain1 : Gain  Gain=I
  Gain2 : Gain  Gain=D
  Integrator : Integrator
  Sum : Sum  Inputs=++|
  Sum1 : Sum  Inputs=++|
  Out1 : Outport
  wires:
  Derivative/1 -> Sum1/2
  Sum1/1 -> Out1/1
  In1/1 -> Gain/1
  Gain1/1 -> Integrator/1
  Integrator/1 -> Sum/2
  Gain/1 -> Gain1/1, Sum/1
  Gain2/1 -> Derivative/1
  Sum/1 -> Gain2/1, Sum1/1

== system PID_controler/pid9/Subsystem2 ==
  In1 : Inport
  Derivative : Derivative
  Gain : Gain  Gain=P
  Gain1 : Gain  Gain=I
  Gain2 : Gain  Gain=D
  Integrator : Integrator
  Sum : Sum  Inputs=+++
  Out1 : Outport
  wires:
  In1/1 -> Gain/1
  Sum/1 -> Out1/1
  Derivative/1 -> Sum/3
  Gain2/1 -> Derivative/1
  Integrator/1 -> Sum/2
  Gain1/1 -> Integrator/1
  Gain/1 -> Sum/1, Gain1/1, Gain2/1
